simulink model "chap12_4sim"  (Simulink 8.3)
settings: Solver=ode45  StartTime=0.0  StopTime=10  FixedStep=0.001  RelTol=1e-3
settings Model: Creator=Administrator  LastModifiedBy=Administrator  ExtModeTrigMode=oneshot  ExtModeArmWhenConnect=off
settings DataIOCC: LimitDataPoints=off  SignalLoggingName=sigsOut
settings OptimizationCC: BooleanDataType=off  ExpressionDepthLimit=2147483647
settings DebuggingCC: SaveWithParameterizedLinksMsg=none  SignalResolutionControl=TryResolveAllWithWarning  SolverPrmCheckMsg=none  MultiTaskDSMMsg=warning  MultiTaskCondExecSysMsg=none  FcnCallInpInsideContextMsg=UseLocalSettings
settings HardwareCC: TargetUnknown=on
settings RTWCC: IncludeERTFirstTime=on

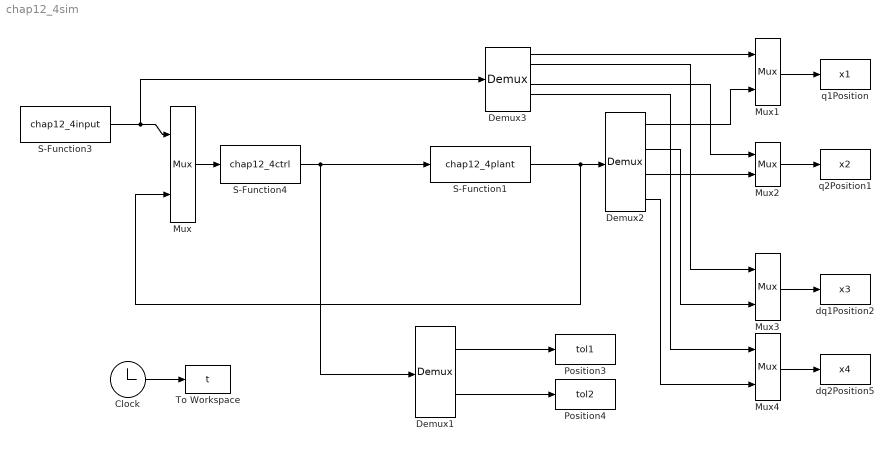
== system chap12_4sim ==
  Clock : Clock
  Demux1 : Demux  Outputs=2
  Demux2 : Demux
  Demux3 : Demux  Outputs=6
  Mux{,1..4} (5 alike) : Mux  Inputs=2
  Position3 : ToWorkspace  VariableName=tol1  SampleTime=-1
  Position4 : ToWorkspace  VariableName=tol2  SampleTime=-1
  S-Function1 : S-Function  FunctionName=chap12_4plant  EnableBusSupport=off
  S-Function3 : S-Function  FunctionName=chap12_4input  EnableBusSupport=off
  S-Function4 : S-Function  FunctionName=chap12_4ctrl  EnableBusSupport=off
  To Workspace : ToWorkspace  VariableName=t  SampleTime=-1
  dq1Position2 : ToWorkspace  VariableName=x3  SampleTime=-1
  dq2Position5 : ToWorkspace  VariableName=x4  SampleTime=-1
  q1Position : ToWorkspace  VariableName=x1  SampleTime=-1
  q2Position1 : ToWorkspace  VariableName=x2  SampleTime=-1
  wires:
  Demux2/1 -> Mux1/2
  S-Function1/1 -> Demux2/1, Mux/2
  Demux1/1 -> Position3/1
  Demux1/2 -> Position4/1
  Demux3/1 -> Mux1/1
  Mux1/1 -> q1Position/1
  Mux2/1 -> q2Position1/1
  Demux3/4 -> Mux2/1
  Clock/1 -> To Workspace/1
  S-Function3/1 -> Mux/1, Demux3/1
  Mux/1 -> S-Function4/1
  S-Function4/1 -> S-Function1/1, Demux1/1
  Demux2/3 -> Mux2/2
  Demux3/2 -> Mux3/1
  Demux2/2 -> Mux3/2
  Demux3/5 -> Mux4/1
  Demux2/4 -> Mux4/2
  Mux3/1 -> dq1Position2/1
  Mux4/1 -> dq2Position5/1
